simulink subsystem "F2ph_to_F3ph"  (R2020a)
settings: Solver=VariableStepAuto  StartTime=0.0  StopTime=10.0  RelTol=1e-3
settings Model: Creator=Nathan Petersen  LastModifiedBy=Nathan Petersen

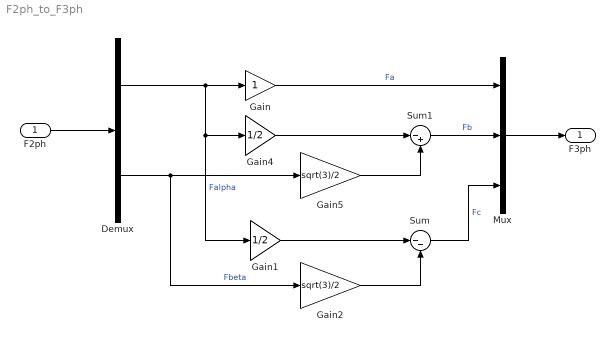
== system F2ph_to_F3ph ==
  F2ph : Inport  PortDimensions=2
  Demux : Demux  Outputs=2
  Gain : Gain
  Gain1 : Gain  Gain=1/2
  Gain2 : Gain  Gain=sqrt(3)/2
  Gain4 : Gain  Gain=1/2
  Gain5 : Gain  Gain=sqrt(3)/2
  Mux : Mux  Inputs=3
  Sum : Sum  Inputs=|--
  Sum1 : Sum  Inputs=|-+
  F3ph : Outport  PortDimensions=3
  wires:
  Demux/2 -> Gain2/1, Gain5/1  "Fbeta"
  Gain5/1 -> Sum1/2
  Gain4/1 -> Sum1/1
  Demux/1 -> Gain1/1, Gain4/1, Gain/1  "Falpha"
  F2ph/1 -> Demux/1
  Sum/1 -> Mux/3  "Fc"
  Gain1/1 -> Sum/1
  Mux/1 -> F3ph/1
  Gain2/1 -> Sum/2
  Sum1/1 -> Mux/2  "Fb"
  Gain/1 -> Mux/1  "Fa"
